simulink model "Model_1"  (R2018b)
settings: Solver=VariableStepDiscrete  StartTime=0.0  StopTime=10.0  MaxStep=0.001  RelTol=1e-3
settings Model: Creator=123  LastModifiedBy=123

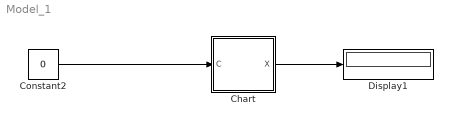
== system Model_1 ==
  Chart : Stateflow chart  TreatAsAtomicUnit=on
  Constant2 : Constant  Value=0
  Display1 : Display
  wires:
  Constant2/1 -> Chart/1(C)
  Chart/1(X) -> Display1/1

== stateflow chart Model_1/Chart ==
  state B
    en:
    X=4;
  state A1
    en:
    X=1;
    du:
    X=2;
    ex:
    X=3;
  (default) -> A1
  A1 -> B : [C==3]
  B -> A1
  data: X output; C input
  events: event local FUNCTION_CALL_EVENT
